simulink model "run_quadrotor_2020a_v2"  (R2020a)
settings: Solver=VariableStepAuto  StartTime=0.0  StopTime=10.0  RelTol=1e-3
InitFcn:
  | fprintf("InitFnc");
  | addpath('display/')
  | addpath('parameters/')
  | addpath('quadrotor_model')
  | addpath('tools/')
  | addpath('libs/RealTime_Pacer')
  | aerosonde_parameters
  | simulation_parameters
  | handles = []
StartFcn:
  | fprintf("StartFnc");
undefined symbols (not defined in the file or in its folder): drawQuadrotor, plotmavstatevariables
libraries: simulink x9
settings Model: Creator=andrey  LastModifiedBy=andrey

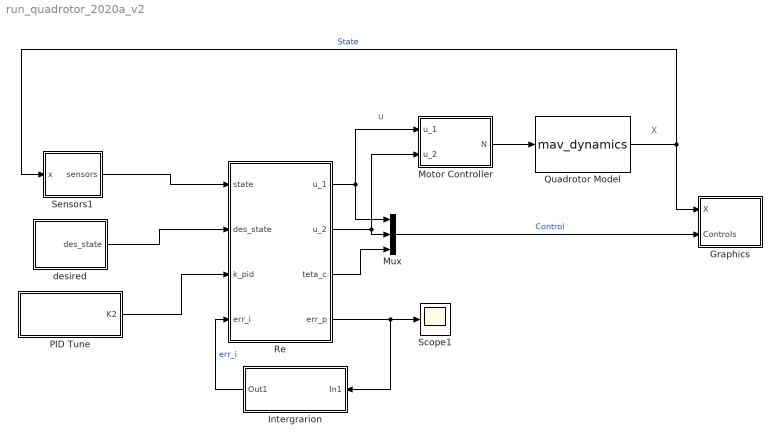
== system run_quadrotor_2020a_v2 ==
  note: u
  note: X
  Graphics : Subsystem
  Intergrarion : Subsystem
  Motor Controller : MATLAB Function  TreatAsAtomicUnit=on
  Mux : Mux  Inputs=3
  PID Tune : Subsystem
  Quadrotor Model : S-Function  FunctionName=mav_dynamics  Parameters=MAV  SFunctionDeploymentMode=off  EnableBusSupport=off
  Re : MATLAB Function  TreatAsAtomicUnit=on
  Scope1 : Scope
  Sensors1 : Subsystem
  desired : MATLAB Function  TreatAsAtomicUnit=on
  wires:
  Mux/1 -> Graphics/2(Controls)  "Control"
  Motor Controller/1(N) -> Quadrotor Model/1
  Intergrarion/1(Out1) -> Re/4(err_i)  "err_i"
  Re/2(u_2) -> Motor Controller/2(u_2), Mux/2
  Re/4(err_p) -> Intergrarion/1(In1), Scope1/1
  Sensors1/1(sensors) -> Re/1(state)
  desired/1(des_state) -> Re/2(des_state)
  Re/1(u_1) -> Motor Controller/1(u_1), Mux/1
  Quadrotor Model/1 -> Graphics/1(X), Sensors1/1("x ")  "State"
  Re/3(teta_c) -> Mux/3
  PID Tune/1(K2) -> Re/3(k_pid)

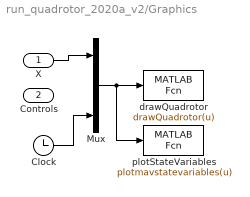
== system run_quadrotor_2020a_v2/Graphics ==
  X : Inport
  Controls : Inport  Port=2
  Clock : Clock
  Mux : Mux  Inputs=3
  drawQuadrotor : MATLABFcn  MATLABFcn=drawQuadrotor(u)  OutputDimensions=0  SampleTime=0.1
  plotStateVariables : MATLABFcn  MATLABFcn=plotmavstatevariables(u)  OutputDimensions=0
  wires:
  X/1 -> Mux/1
  Mux/1 -> plotStateVariables/1, drawQuadrotor/1
  Clock/1 -> Mux/3

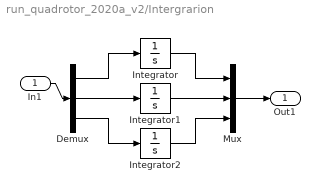
== system run_quadrotor_2020a_v2/Intergrarion ==
  In1 : Inport
  Demux : Demux  Outputs=3
  Integrator : Integrator
  Integrator1 : Integrator
  Integrator2 : Integrator
  Mux : Mux  Inputs=3
  Out1 : Outport
  wires:
  In1/1 -> Demux/1
  Mux/1 -> Out1/1
  Integrator/1 -> Mux/1
  Integrator1/1 -> Mux/2
  Integrator2/1 -> Mux/3
  Demux/3 -> Integrator2/1
  Demux/2 -> Integrator1/1
  Demux/1 -> Integrator/1

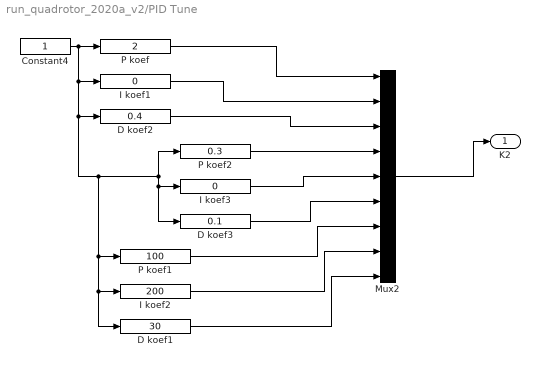
== system run_quadrotor_2020a_v2/PID Tune ==
  Constant4 : Constant
  D koef1 : simulink/Math Operations/Slider Gain  gain=30  low=0  high=5000
  D koef2 : simulink/Math Operations/Slider Gain  gain=0.4  low=0  high=5000
  D koef3 : simulink/Math Operations/Slider Gain  gain=0.1  low=0  high=5000
  I koef1 : simulink/Math Operations/Slider Gain  gain=0  low=0  high=5000
  I koef2 : simulink/Math Operations/Slider Gain  gain=200  low=0  high=5000
  I koef3 : simulink/Math Operations/Slider Gain  gain=0  low=0  high=5000
  Mux2 : Mux  Inputs=9
  P koef : simulink/Math Operations/Slider Gain  gain=2  low=0  high=30000
  P koef1 : simulink/Math Operations/Slider Gain  gain=100  low=0  high=30000
  P koef2 : simulink/Math Operations/Slider Gain  gain=0.3  low=0  high=30000
  K2 : Outport
  wires:
  Mux2/1 -> K2/1
  Constant4/1 -> I koef1/1, I koef2/1, D koef1/1, P koef1/1, P koef2/1, I koef3/1, D koef3/1, D koef2/1, P koef/1
  P koef/1 -> Mux2/1
  I koef1/1 -> Mux2/2
  D koef2/1 -> Mux2/3
  P koef2/1 -> Mux2/4
  I koef3/1 -> Mux2/5
  D koef3/1 -> Mux2/6
  P koef1/1 -> Mux2/7
  I koef2/1 -> Mux2/8
  D koef1/1 -> Mux2/9

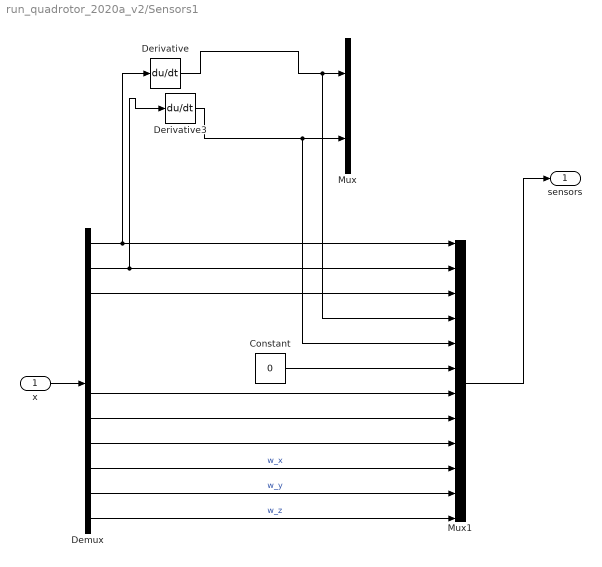
== system run_quadrotor_2020a_v2/Sensors1 ==
  "x " : Inport
  Constant : Constant  Value=0
  Demux : Demux  Outputs=12
  Derivative : Derivative
  Derivative3 : Derivative
  Mux : Mux  Inputs=2
  Mux1 : Mux  Inputs=12
  sensors : Outport
  wires:
  "x "/1 -> Demux/1
  Derivative/1 -> Mux1/4, Mux/1
  Demux/2 -> Derivative3/1, Mux1/2
  Derivative3/1 -> Mux1/5, Mux/2
  Demux/1 -> Derivative/1, Mux1/1
  Demux/3 -> Mux1/3
  Constant/1 -> Mux1/6
  Demux/12 -> Mux1/12  "w_z"
  Demux/11 -> Mux1/11  "w_y"
  Demux/10 -> Mux1/10  "w_x"
  Demux/9 -> Mux1/9
  Demux/8 -> Mux1/8
  Demux/7 -> Mux1/7
  Mux1/1 -> sensors/1

== matlab function run_quadrotor_2020a_v2/Re ==
  data: u_1 output; u_2 output; teta_c output; state input; des_state input; k_pid input; err_p output; err_i input size=3
function [u_1, u_2, teta_c, err_p] = fcn(state, des_state, k_pid, err_i)
    % код регулятора вынесен в .mat файл, чтобы корректно отображался в
    % git-истории
    [teta_c, u_1, u_2, err_p] = regul(state, des_state, k_pid, err_i);

== matlab function run_quadrotor_2020a_v2/Motor Controller ==
  data: N output; u_1 input; u_2 input
function N = fcn(u_1, u_2)

% teta_c = data(1);
% u_1 = data(2);
% u_2 = data(3);

NN = 0.25*[u_1+u_2 u_1+u_2 u_1-u_2 u_1-u_2]';
N = sqrt(NN);

== matlab function run_quadrotor_2020a_v2/desired ==
  data: des_state output
function des_state = fcn()

pos = [1 0 0]';
vel = [0 0 0]';
acc = [0 0 0]';
des_state = [pos vel acc];
